simulink model "old_envModel_rl"  (R2020b)
settings: Solver=ode23t  StartTime=0.0  StopTime=8  RelTol=1e-2
values from neighbouring files (symbols this model uses):
  simlen = 80    [new_main_rl.m]    (also in old_main_rl.m = 5)
  Tf = simlen*Ts    [new_main_rl.m]    (also in old_main_rl.m)
  Ts = s.Ts    [new_main_rl.m]    (also in old_main_rl.m)
  ulim = s.actuatorRange    [new_main_rl.m]    (also in old_main_rl.m)
  whichAg_sim = whichAg_sim*5    (= 30)    [new_main_rl.m]    (also in old_main_rl.m)
  ylim = s.sensorRange    [new_main_rl.m]    (also in old_main_rl.m)
undefined symbols (not defined in the file or in its folder): s
libraries: rllib x3, simulink x2
settings Model: Creator=The MathWorks, Inc.  LastModifiedBy=user
settings DataIOCC: ExternalInput=s  SaveFormat=Structure  SaveOutput=off  SignalLogging=off  InspectSignalLogs=on  SaveTime=off  DSMLoggingName=s

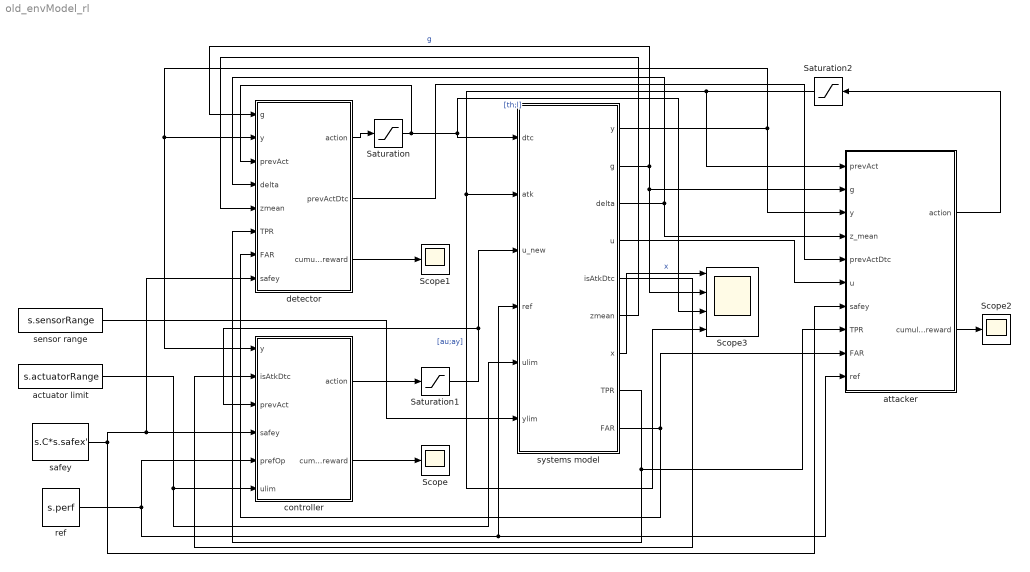
== system old_envModel_rl ==
  Saturation : Saturate  UpperLimit=[100;simlen]  LowerLimit=[0;1]
  Saturation1 : Saturate  UpperLimit=s.actuatorRange  LowerLimit=-s.actuatorRange
  Saturation2 : Saturate  UpperLimit=[ulim;ylim]  LowerLimit=-[ulim;ylim]
  Scope : Scope
  Scope1 : Scope
  Scope2 : Scope
  Scope3 : Scope  NumInputPorts=4
  actuator limit : Constant  Value=s.actuatorRange
  attacker : Subsystem
  controller : Subsystem
  detector : Subsystem
  ref : Constant  Value=s.perf
  safey : Constant  Value=s.C*s.safex'
  sensor range : Constant  Value=s.sensorRange
  systems model : Subsystem
  wires:
  systems model/1(y) -> detector/2(y), controller/1(y), attacker/3(y)
  ref/1 -> attacker/10(ref), systems model/4(ref), controller/5(prefOp)
  safey/1 -> attacker/7(safey), detector/8(safey), controller/4(safey)
  systems model/3(delta) -> detector/4(delta), attacker/4(z_mean)
  systems model/2(g) -> detector/1(g), Scope3/2, attacker/2(g)  "g"
  sensor range/1 -> systems model/6(ylim)
  actuator limit/1 -> systems model/5(ulim), controller/6(ulim)
  Saturation/1 -> detector/3(prevAct), Scope3/3, systems model/1(dtc)  "[th;l]"
  Saturation1/1 -> systems model/3(u_new), controller/3(prevAct)
  Saturation2/1 -> attacker/1(prevAct), Scope3/4, systems model/2(atk)  "[au;ay]"
  systems model/7(x) -> Scope3/1  "x"
  systems model/9(FAR) -> attacker/9(FAR), detector/7(FAR)
  systems model/8(TPR) -> attacker/8(TPR), detector/6(TPR)
  systems model/6(zmean) -> detector/5(zmean)
  detector/1(action) -> Saturation/1
  detector/3(cumulative_reward) -> Scope1/1
  systems model/5(isAtkDtc) -> controller/2(isAtkDtc)
  controller/1(action) -> Saturation1/1
  controller/2(cumulative_reward) -> Scope/1
  detector/2(prevActDtc) -> attacker/5(prevActDtc)
  systems model/4(u) -> attacker/6(u)
  attacker/1(action) -> Saturation2/1
  attacker/2(cumulative_reward) -> Scope2/1

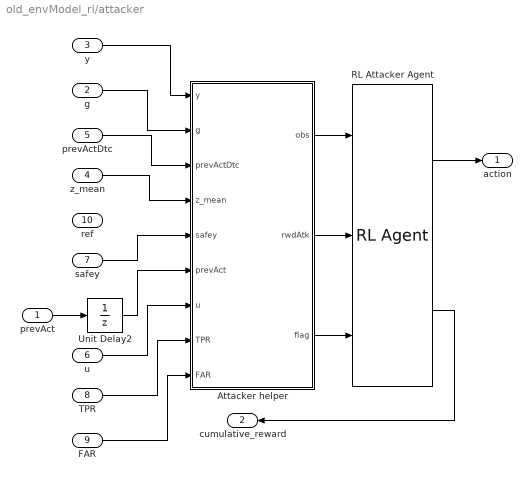
== system old_envModel_rl/attacker ==
  prevAct : Inport
  g : Inport  Port=2
  y : Inport  Port=3
  z_mean : Inport  Port=4
  prevActDtc : Inport  Port=5
  u : Inport  Port=6
  safey : Inport  Port=7
  TPR : Inport  Port=8
  FAR : Inport  Port=9
  ref : Inport  Port=10
  Attacker helper : Subsystem
  RL Attacker Agent : rllib/RL Agent  Agent=agentAtk  ProvideReward=on  ProvideIsDone=on  ProvideCumRwd=on  TreatAsDirectFeedthrough=on  CollectLoggedSignals=on  CollectModelStates=on
  Unit Delay2 : UnitDelay  SampleTime=-1  HasFrameUpgradeWarning=on
  action : Outport
  cumulative_reward : Outport  Port=2
  wires:
  z_mean/1 -> Attacker helper/4(z_mean)
  prevAct/1 -> Unit Delay2/1
  y/1 -> Attacker helper/1(y)
  Attacker helper/3(flag) -> RL Attacker Agent/3
  Attacker helper/1(obs) -> RL Attacker Agent/1
  Attacker helper/2(rwdAtk) -> RL Attacker Agent/2
  RL Attacker Agent/2 -> cumulative_reward/1
  Unit Delay2/1 -> Attacker helper/6(prevAct)
  RL Attacker Agent/1 -> action/1
  TPR/1 -> Attacker helper/8(TPR)
  FAR/1 -> Attacker helper/9(FAR)
  prevActDtc/1 -> Attacker helper/3(prevActDtc)
  g/1 -> Attacker helper/2(g)
  u/1 -> Attacker helper/7(u)
  safey/1 -> Attacker helper/5(safey)

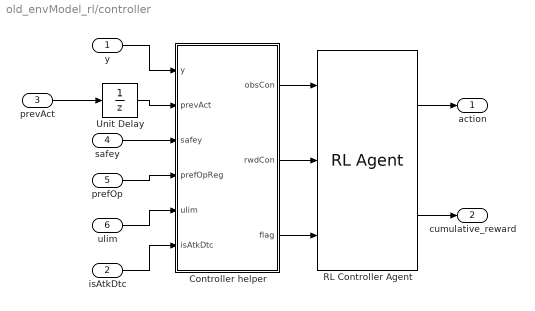
== system old_envModel_rl/controller ==
  y : Inport
  isAtkDtc : Inport  Port=2
  prevAct : Inport  Port=3
  safey : Inport  Port=4
  prefOp : Inport  Port=5
  ulim : Inport  Port=6
  Controller helper : Subsystem
  RL Controller Agent : rllib/RL Agent  Agent=agentCon  ProvideReward=on  ProvideIsDone=on  ProvideCumRwd=on  TreatAsDirectFeedthrough=on  CollectLoggedSignals=on  CollectModelStates=on
  Unit Delay : UnitDelay  SampleTime=-1  HasFrameUpgradeWarning=on
  action : Outport
  cumulative_reward : Outport  Port=2
  wires:
  Unit Delay/1 -> Controller helper/2(prevAct)
  RL Controller Agent/2 -> cumulative_reward/1
  prefOp/1 -> Controller helper/4(prefOpReg)
  Controller helper/1(obsCon) -> RL Controller Agent/1
  ulim/1 -> Controller helper/5(ulim)
  Controller helper/3(flag) -> RL Controller Agent/3
  safey/1 -> Controller helper/3(safey)
  prevAct/1 -> Unit Delay/1
  Controller helper/2(rwdCon) -> RL Controller Agent/2
  isAtkDtc/1 -> Controller helper/6(isAtkDtc)
  RL Controller Agent/1 -> action/1
  y/1 -> Controller helper/1(y)

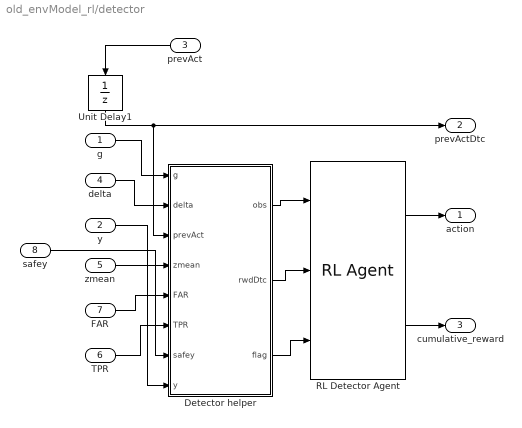
== system old_envModel_rl/detector ==
  g : Inport
  y : Inport  Port=2
  prevAct : Inport  Port=3
  delta : Inport  Port=4
  zmean : Inport  Port=5
  TPR : Inport  Port=6
  FAR : Inport  Port=7
  safey : Inport  Port=8
  Detector helper : Subsystem
  RL Detector Agent : rllib/RL Agent  Agent=agentDtc  ProvideReward=on  ProvideIsDone=on  ProvideCumRwd=on  TreatAsDirectFeedthrough=on  CollectLoggedSignals=on  CollectModelStates=on
  Unit Delay1 : UnitDelay  SampleTime=-1  HasFrameUpgradeWarning=on
  action : Outport
  prevActDtc : Outport  Port=2
  cumulative_reward : Outport  Port=3
  wires:
  FAR/1 -> Detector helper/5(FAR)
  TPR/1 -> Detector helper/6(TPR)
  g/1 -> Detector helper/1(g)
  prevAct/1 -> Unit Delay1/1
  RL Detector Agent/2 -> cumulative_reward/1
  Detector helper/3(flag) -> RL Detector Agent/3
  Detector helper/1(obs) -> RL Detector Agent/1
  Detector helper/2(rwdDtc) -> RL Detector Agent/2
  RL Detector Agent/1 -> action/1
  zmean/1 -> Detector helper/4(zmean)
  delta/1 -> Detector helper/2(delta)
  Unit Delay1/1 -> prevActDtc/1, Detector helper/3(prevAct)
  y/1 -> Detector helper/8(y)
  safey/1 -> Detector helper/7(safey)

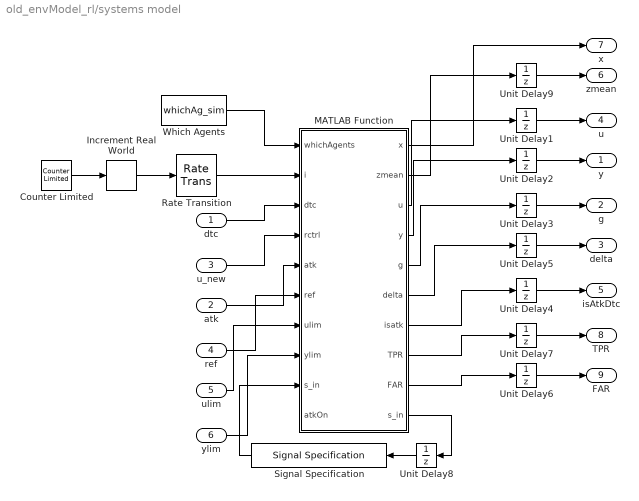
== system old_envModel_rl/systems model ==
  dtc : Inport
  atk : Inport  Port=2
  u_new : Inport  Port=3
  ref : Inport  Port=4
  ulim : Inport  Port=5
  ylim : Inport  Port=6
  Counter Limited : simulink/Sources/Counter Limited  uplimit=Tf/Ts-2  tsamp=Ts
  Increment Real World : simulink/Additional Math & Discrete/Additional Math: Increment - Decrement/Increment Real World
      settings: SourceProductBaseCode=SL
  MATLAB Function : MATLAB Function  TreatAsAtomicUnit=on
  Rate Transition : RateTransition
  Signal Specification : SignalSpecification  OutDataTypeStr=Bus: slBus1  BusOutputAsStruct=on
  Unit Delay{1..7,9} (8 alike) : UnitDelay  SampleTime=-1  HasFrameUpgradeWarning=on
  Unit Delay8 : UnitDelay  InitialCondition=s  SampleTime=-1  HasFrameUpgradeWarning=on
  Which Agents : Constant  Value=whichAg_sim  SampleTime=Ts
  y : Outport
  g : Outport  Port=2
  delta : Outport  Port=3
  u : Outport  Port=4
  isAtkDtc : Outport  Port=5
  zmean : Outport  Port=6
  x : Outport  Port=7
  TPR : Outport  Port=8
  FAR : Outport  Port=9
  wires:
  Unit Delay9/1 -> zmean/1
  Unit Delay7/1 -> TPR/1
  Unit Delay6/1 -> FAR/1
  Unit Delay2/1 -> y/1
  MATLAB Function/8(TPR) -> Unit Delay7/1
  Unit Delay3/1 -> g/1
  Unit Delay4/1 -> isAtkDtc/1
  Unit Delay5/1 -> delta/1
  Increment Real World/1 -> Rate Transition/1
  Rate Transition/1 -> MATLAB Function/2(i)
  MATLAB Function/5(g) -> Unit Delay3/1
  MATLAB Function/6(delta) -> Unit Delay5/1
  ulim/1 -> MATLAB Function/7(ulim)
  Which Agents/1 -> MATLAB Function/1(whichAgents)
  MATLAB Function/4(y) -> Unit Delay2/1
  Unit Delay1/1 -> u/1
  ref/1 -> MATLAB Function/6(ref)
  ylim/1 -> MATLAB Function/8(ylim)
  Counter Limited/1 -> Increment Real World/1
  MATLAB Function/3(u) -> Unit Delay1/1
  atk/1 -> MATLAB Function/5(atk)
  dtc/1 -> MATLAB Function/3(dtc)
  MATLAB Function/7(isatk) -> Unit Delay4/1
  u_new/1 -> MATLAB Function/4(rctrl)
  MATLAB Function/1(x) -> x/1
  MATLAB Function/2(zmean) -> Unit Delay9/1
  MATLAB Function/9(FAR) -> Unit Delay6/1
  MATLAB Function/10(s_in) -> Unit Delay8/1
  Signal Specification/1 -> MATLAB Function/9("s_in ")
  Unit Delay8/1 -> Signal Specification/1

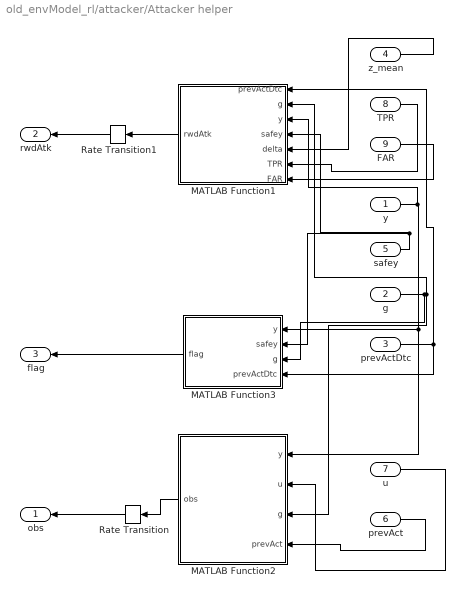
== system old_envModel_rl/attacker/Attacker helper ==
  y : Inport
  g : Inport  Port=2
  prevActDtc : Inport  Port=3
  z_mean : Inport  Port=4
  safey : Inport  Port=5
  prevAct : Inport  Port=6
  u : Inport  Port=7
  TPR : Inport  Port=8
  FAR : Inport  Port=9
  MATLAB Function1 : MATLAB Function  TreatAsAtomicUnit=on
  MATLAB Function2 : MATLAB Function  TreatAsAtomicUnit=on
  MATLAB Function3 : MATLAB Function  TreatAsAtomicUnit=on
  Rate Transition : RateTransition
  Rate Transition1 : RateTransition
  obs : Outport
  rwdAtk : Outport  Port=2
  flag : Outport  Port=3
  wires:
  MATLAB Function1/1(rwdAtk) -> Rate Transition1/1
  z_mean/1 -> MATLAB Function1/5(delta)
  prevAct/1 -> MATLAB Function2/4(prevAct)
  u/1 -> MATLAB Function2/2(u)
  TPR/1 -> MATLAB Function1/6(TPR)
  MATLAB Function3/1(flag) -> flag/1
  FAR/1 -> MATLAB Function1/7(FAR)
  Rate Transition/1 -> obs/1
  safey/1 -> MATLAB Function1/4(safey), MATLAB Function3/2(safey)
  MATLAB Function2/1(obs) -> Rate Transition/1
  Rate Transition1/1 -> rwdAtk/1
  prevActDtc/1 -> MATLAB Function3/4(prevActDtc), MATLAB Function1/1(prevActDtc)
  y/1 -> MATLAB Function2/1(y), MATLAB Function3/1(y), MATLAB Function1/3(y)
  g/1 -> MATLAB Function2/3(g), MATLAB Function1/2(g), MATLAB Function3/3(g)

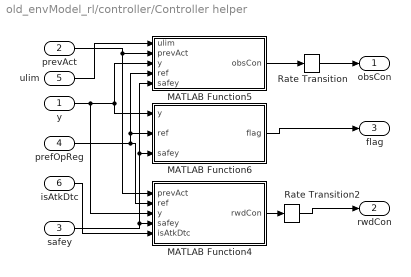
== system old_envModel_rl/controller/Controller helper ==
  y : Inport
  prevAct : Inport  Port=2
  safey : Inport  Port=3
  prefOpReg : Inport  Port=4
  ulim : Inport  Port=5
  isAtkDtc : Inport  Port=6
  MATLAB Function4 : MATLAB Function  TreatAsAtomicUnit=on
  MATLAB Function5 : MATLAB Function  TreatAsAtomicUnit=on
  MATLAB Function6 : MATLAB Function  TreatAsAtomicUnit=on
  Rate Transition : RateTransition
  Rate Transition2 : RateTransition
  obsCon : Outport
  rwdCon : Outport  Port=2
  flag : Outport  Port=3
  wires:
  prefOpReg/1 -> MATLAB Function6/2(ref), MATLAB Function5/4(ref), MATLAB Function4/2(ref)
  safey/1 -> MATLAB Function5/5(safey), MATLAB Function6/3(safey), MATLAB Function4/4(safey)
  MATLAB Function4/1(rwdCon) -> Rate Transition2/1
  MATLAB Function5/1(obsCon) -> Rate Transition/1
  y/1 -> MATLAB Function6/1(y), MATLAB Function5/3(y), MATLAB Function4/3(y)
  prevAct/1 -> MATLAB Function4/1(prevAct), MATLAB Function5/2(prevAct)
  Rate Transition/1 -> obsCon/1
  MATLAB Function6/1(flag) -> flag/1
  ulim/1 -> MATLAB Function5/1(ulim)
  Rate Transition2/1 -> rwdCon/1
  isAtkDtc/1 -> MATLAB Function4/5(isAtkDtc)

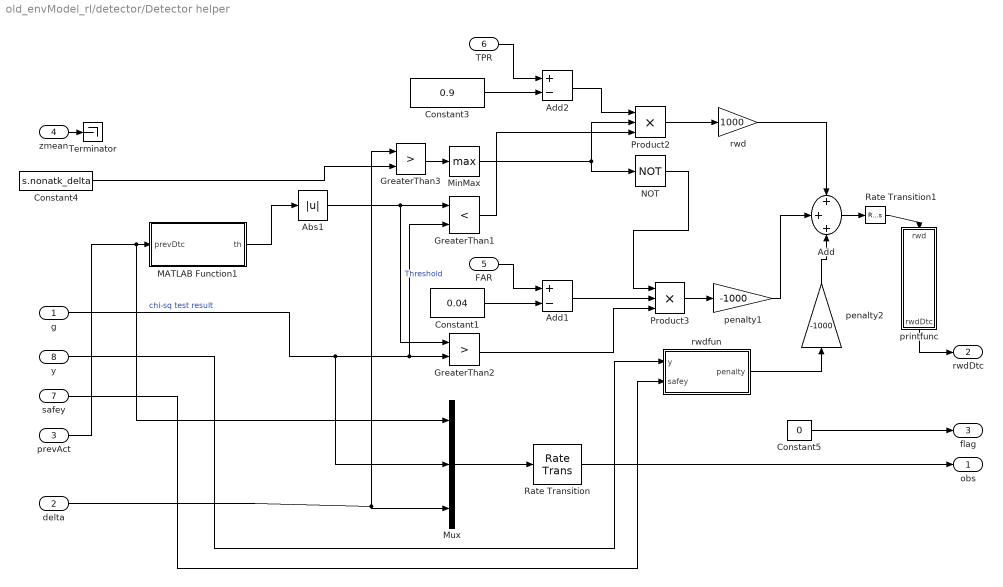
== system old_envModel_rl/detector/Detector helper ==
  g : Inport
  delta : Inport  Port=2
  prevAct : Inport  Port=3
  zmean : Inport  Port=4
  FAR : Inport  Port=5
  TPR : Inport  Port=6
  safey : Inport  Port=7
  y : Inport  Port=8
  " printfunc" : MATLAB Function  TreatAsAtomicUnit=on
  Abs1 : Abs
  Add : Sum  Inputs=+++
  Add1 : Sum  Inputs=+-
  Add2 : Sum  Inputs=+-
  Constant1 : Constant  Value=0.04  SampleTime=Ts
  Constant3 : Constant  Value=0.9  SampleTime=Ts
  Constant4 : Constant  Value=s.nonatk_delta  SampleTime=Ts
  Constant5 : Constant  Value=0  SampleTime=Ts
  GreaterThan1 : RelationalOperator  Operator=<  OutDataTypeStr=boolean  RndMeth=Simplest
  GreaterThan2 : RelationalOperator  Operator=>  OutDataTypeStr=boolean  RndMeth=Simplest
  GreaterThan3 : RelationalOperator  Operator=>  OutDataTypeStr=boolean  RndMeth=Simplest
  MATLAB Function1 : MATLAB Function  TreatAsAtomicUnit=on
  MinMax : MinMax  Function=max
  Mux : Mux  Inputs=3
  NOT : Logic  Operator=NOT  IconShape=distinctive  AllPortsSameDT=off  OutDataTypeStr=boolean
  Product2 : Product  Inputs=3
  Product3 : Product  Inputs=3
  Rate Transition : RateTransition
  Rate Transition1 : RateTransition
  Terminator : Terminator
  penalty1 : Gain  Gain=-1000
  penalty2 : Gain  Gain=-1000
  rwd : Gain  Gain=1000
  rwdfun : MATLAB Function  TreatAsAtomicUnit=on
  obs : Outport
  rwdDtc : Outport  Port=2
  flag : Outport  Port=3
  wires:
  GreaterThan1/1 -> Product2/3
  GreaterThan2/1 -> Product3/3
  NOT/1 -> Product3/1
  Constant5/1 -> flag/1
  Product3/1 -> penalty1/1
  Abs1/1 -> GreaterThan1/1, GreaterThan2/1  "Threshold"
  Add1/1 -> Product3/2
  Add2/1 -> Product2/1
  Product2/1 -> rwd/1
  Rate Transition/1 -> obs/1
  Constant3/1 -> Add2/2
  prevAct/1 -> Mux/1, MATLAB Function1/1(prevDtc)
  Mux/1 -> Rate Transition/1
  " printfunc"/1(rwdDtc) -> rwdDtc/1
  Constant1/1 -> Add1/2
  TPR/1 -> Add2/1
  FAR/1 -> Add1/1
  MATLAB Function1/1(th) -> Abs1/1
  rwd/1 -> Add/1
  GreaterThan3/1 -> MinMax/1
  g/1 -> Mux/2, GreaterThan2/2, GreaterThan1/2  "chi-sq test result"
  penalty1/1 -> Add/2
  Constant4/1 -> GreaterThan3/2
  MinMax/1 -> NOT/1, Product2/2
  delta/1 -> GreaterThan3/1, Mux/3
  zmean/1 -> Terminator/1
  Add/1 -> Rate Transition1/1
  Rate Transition1/1 -> " printfunc"/1(rwd)
  y/1 -> rwdfun/1(y)
  safey/1 -> rwdfun/2(safey)
  rwdfun/1(penalty) -> penalty2/1
  penalty2/1 -> Add/3

== matlab function old_envModel_rl/controller/Controller helper/MATLAB Function5 ==
  data: ulim input; obsCon output; prevAct input; y input; ref input; safey input
function obsCon = obsCon(ulim,prevAct,y,ref,safey)
   
    obsCon=[ulim;prevAct;y;ref;safey];

== matlab function old_envModel_rl/controller/Controller helper/MATLAB Function6 ==
  data: y input; ref input; flag output; safey input
function flag = stop(y,ref,safey)
flag= 0;
% flag = abs((y-ref)/ref) <= 0.25;

== matlab function old_envModel_rl/detector/Detector helper/ printfunc ==
  data: rwd input; rwdDtc output
function rwdDtc = printVal(rwd)
rwdDtc = rwd

== matlab function old_envModel_rl/detector/Detector helper/MATLAB Function1 ==
  data: prevDtc input; th output
function th   = split(prevDtc)
%    format long g;
   th = prevDtc(1);
    l = prevDtc(2);
end

== matlab function old_envModel_rl/detector/Detector helper/rwdfun ==
  data: y input; penalty output; safey input
function penalty = penY(y,safey)
penalty = max(abs(y)-abs(safey))/max(safey);

== matlab function old_envModel_rl/attacker/Attacker helper/MATLAB Function1 ==
  data: rwdAtk output; prevActDtc input; g input; y input; safey input; delta input; TPR input; FAR input
function rwdAtk  = rwrdAtk(prevActDtc,g,y,safey,delta,TPR,FAR)
%    format long g;
   th = abs(prevActDtc(1));
   tau = max(1,ceil(prevActDtc(2,1)));
   dof = size(y,1)*(tau);
%    FAR = chi2cdf(th,dof,'upper')
%    TPR = ncx2cdf(th,dof,abs(delta),'upper');
%    rwdAtk = FAR/TPR + 50*(g<th)+ 100*(y-ref)^2;
%             50*(FAR-0.05)-40*TPR + 50*(g<th)+ 100*(abs(y)-abs(safey))
% % rwdAtk = 50*(1-FAR) -50*TPR + 100*(g<th & abs(y)>abs(safey))+ 100*(abs(y)-abs(safey))
% rwdAtk = 50*(-FAR) -50*TPR + 100*(g<th)*(abs(y)-abs(safey))+ 100*(g<th)*(abs(y)-0.4*abs(safey))
rwdAtk = 500*(FAR) -1000*TPR + 1000*(g<=th)*max(abs(y)-abs(safey))/max(abs(safey))+1000*(th<=g)

== matlab function old_envModel_rl/systems model/MATLAB Function ==
  data: x output; zmean output; whichAgents input; u output; i input; y output; g output; delta output; dtc input; rctrl input; atk input; ref input; ulim input; ylim input; isatk output; TPR output; FAR output; s_in output; s_in input Bus: slBus1; atkOn input
function [x,zmean,u,y,g,delta,isatk,TPR,FAR,s_in] = env(whichAgents,i,dtc,rctrl,atk,ref,ulim,ylim,s_in, atkOn)
% function [y,g,z_mean]= envSys(atk,dtc,new_u,ref, s)
disp("-------------iteration: "+i+"--------------")
xdim= size(s_in.A,2);
ydim= size(s_in.C,1);
udim= size(s_in.B,2);
au= zeros(udim,1);
ay= zeros(ydim,1);
%% SYS_ENV progress every iteration goes here
if ~rem(whichAgents,2)
    disp("with attacker agent");
    for i1=1:udim
        au(i1,1)= atk(i1,1);
    end
    for i2=1:udim
        ay(i2,1)= atk(udim+i2,1);
    end  
else
    disp("without attacker agent, no attack");
    au=zeros(udim,1);
    ay=zeros(ydim,1);
end
if ~atkOn
    disp(" no attack FAR test");
    au=zeros(udim,1);
    ay=zeros(ydim,1);
end
% % 3 for controller agent % added later durng detection
% if ~rem(whichAgents,3)
%     u_new= rctrl;
%     disp("with controller agent");
% else
%     u_new = zeros(size(rctrl));
%     disp("without controller agent, with default control action");
% end
% 5 for detector agent
if ~rem(whichAgents,5)
    th= abs(dtc(1));
    dtc_windw= max(1,(ceil(dtc(2))));
%     prevDtc = dtc;
    disp("with detector agent");
else
    disp("without detector agent, with default threshold, dof");
    th=s_in.th;
    dtc_windw=1;
%     prevDtc= [th;dtc_windw];
end

%             s_in.t(i+1)=s_in.t(i)+s_in.Ts;

            s_in.a_u(:,i)=au.*s_in.uatkon;

            s_in.a_y(:,i)=ay.*s_in.yatkon;
           
            s_in.est_err(:,i)= s_in.x_act(:,i)-s_in.xhat(:,i);
            
            s_in.u_act(:,i)= max(-ulim,min(ulim,s_in.K*s_in.xhat(:,i)));
            
            s_in.uatk(:,i)= max(-ulim,min(ulim,s_in.u_act(:,i)+s_in.a_u(:,i)));
            
            s_in.y_act(:,i)= max(-ylim,min(ylim,s_in.C*s_in.x_act(:,i))+s_in.meas_noise(:,i));
            
            s_in.yatk(:,i)= max(-ylim,min(ylim,s_in.y_act(:,i)+s_in.a_y(:,i)));
            
            s_in.z(:,i)= s_in.yatk(:,i)-s_in.C*s_in.xhat(:,i);
            
            s_in.x_act(:,i+1) = s_in.A*s_in.x_act(:,i)-s_in.B*s_in.uatk(:,i)+s_in.proc_noise(:,i);

            s_in.xhat(:,i+1) = s_in.A*s_in.xhat(:,i) - s_in.B*s_in.u_act(:,i) + s_in.L*s_in.z(:,i);
%             assignin('base','s_in.xhat', s_in.xhat);
% 3 for controller agent
if ~rem(whichAgents,3)
    u_new= rctrl;
    disp("with controller agent");
else
    u_new = s_in.uatk(:,i);
    disp("without controller agent, with default control action");
end 
%             disp("print check values");
%             au= s_in.a_u
%             ay= s_in.a_y
%             xval= s_in.x_act
%             xhat= s_in.xhat
%             esterr= s_in.est_err
%             uval= s_in.u_act
%             uatk= s_in.uatk
%             yval= s_in.y_act
%             yatk= s_in.yatk
%             Cxhat= s_in.C*s_in.xhat
            
            for i3=1:size(s_in.z,1)
                disp("print: checking mean calc: z_cur, mean,var")
                z_current=s_in.z(i3,1:i)';
                mean(z_current)'
                var(z_current)'
                s_in.z_mean(i3,i)= mean(z_current)';
                s_in.z_var(i3,i) = var(z_current)';
                
            end
            disp("print checking z_val");
%             zval= [s_in.z(1,1:i+1);s_in.z(2,1:i+1)]
            s_in.chi_tst(i)= (s_in.z(:,i)'/s_in.nonatk_zvar)*s_in.z(:,i); % ttc without noise z var=0.1
%             s_in.chi_tst(i+1)= s_in.z(:,i+1)'*inv(cov(s_in.z'))*s_in.z(:,i+1);
%              if ~isfinite(s_in.chi_tst(i))
%                     s_in.chi_tst(i)= 0;
%              end
            s_in.threshold(i)= th;
            s_in.tau(i)= dtc_windw;
            s_in.g(i) = 0;
            s_in.non_cent(:,i)= 0;
%             if i-tau+1 > 0                  % Calculate detector window starting index
%                 srt = i-tau+1;              % tau is the detector window length
%             else
%                 srt = 1;
%             end
            disp("print z_cov");
            z_covar = cov( s_in.z(:,1:i)')
%             if det(z_covar)==0
%                 s_in.z_var(:,i+1)=s_in.z_var(:,i);
%                 disp("singular")
%             end
%             disp("print here");
%% Chi square test and non centrality calculation
            for k = max(1,i-s_in.tau(i)+1):i
                s_in.g(i) = s_in.g(i) + s_in.chi_tst(k);  % Calculate gk (chi2 test)
                currentzmean= s_in.z_mean;
                disp("print checking non_cent");
                del= (s_in.z_mean(:,k)'/z_covar)*s_in.z_mean(:,k)
%                 del= s_in.z_mean(:,k+1)'*inv(cov(s_in.z'))*s_in.z_mean(:,k+1);
                if ~isfinite(del)
                    disp("print adding zero non_cent if value is inf or nan");
                    s_in.non_cent(i)= s_in.non_cent(i) + 0;
                else
                    s_in.non_cent(i)= s_in.non_cent(i) + del;
                    disp("print adding finite non_cent");
                end
            end
            noncent= s_in.non_cent(:,i)
            disp("print chisq test val");
            chitest= s_in.chi_tst(:,i)
            gvals= s_in.g(:,i)
            
%% to start the RL based controller
%             if (max(abs(s_in.yatk(i))>abs(s_in.C*s_in.safex'))) || (s_in.g(i) > s_in.threshold(i))
              if (s_in.g(i) > s_in.threshold(i))
                s_in.u_act(:,i) = max(-ulim,min(ulim,u_new));
                s_in.uatk(:,i)= max(-ulim,min(ulim,s_in.u_act(:,i)+s_in.a_u(:,i)));
                isatk=1;
                disp("detected");
                disp("print  new u");
                newu= s_in.u_act(:,i)
                newuatk= s_in.uatk(:,i)
            else
                isatk=0;
            end
            

    th= s_in.threshold(i)
    window= s_in.tau(i)
    dof= s_in.tau(i)*size(s_in.C,1)
    TPR= ncx2cdf(s_in.threshold(i),dof,s_in.non_cent(i),'upper')
    FAR= chi2cdf(s_in.threshold(i),dof,'upper')
    s_in.avgtpr(i)= TPR;
    s_in.avgfar(i)= FAR;
    avgtpr= mean(s_in.avgtpr)
    avgfar= mean(s_in.avgfar)
    g= s_in.g(i);
    y= s_in.yatk(:,i)
    u= s_in.uatk(:,i)
    delta = s_in.non_cent(i);
    ay_act= ay;
    au_act = au;
%     if (ay == ylim || ay == -ylim)
%         ay_act = ay- s_in.y_act(:,i);
%     end
%     if (au == ulim || au == -ulim)
%         au_act= au- s_in.u_act(:,i);
%     end
    fdi = [ay_act;au_act]
    x= s_in.x_act(:,i);
    zmean= s_in.z_mean(:,i);
%     prevDtc=[s_in.threshold(i);s_in.tau(i)];
end

== matlab function old_envModel_rl/attacker/Attacker helper/MATLAB Function2 ==
  data: obs output; y input; u input; g input; prevAct input
function obs = obsAtk(y,u,g,prevAct)
%     format long g;
    ay= prevAct(1,1);
    au= prevAct(2,1);
    obs= [y;u;g;prevAct];

== matlab function old_envModel_rl/attacker/Attacker helper/MATLAB Function3 ==
  data: y input; flag output; safey input; g input; prevActDtc input
function flag  = stop(y,safey, g, prevActDtc)
%     format long g;
    th = abs(prevActDtc(1));
%     flag = g > th;
flag= 0;

== matlab function old_envModel_rl/controller/Controller helper/MATLAB Function4 ==
  data: rwdCon output; prevAct input; ref input; y input; safey input; isAtkDtc input
function rwdCon  = rwrdCon(prevAct,ref,y,safey,isAtkDtc)
%     format long g;
    u=prevAct;
%     ay=atk(2);
    %% safer : 0.5* safey
%     rwdCon = 350*(abs((y-ref)/ref) <= 0.30)-20*(prevAct)^2-100*(abs(y) > safey)-50
% rwdCon = isAtkDtc*(-(y-ref*safey)'*1000*(y-ref*safey))%-20*u^2
% rwdCon = isAtkDtc*(abs(ref*safey)-abs(y))'*1000*(abs(ref*safey)-abs(y))
rwdCon = isAtkDtc*1000*max(abs(ref*safey)-abs(y))/max(abs(ref*safey))
